simulink model "SPACE584toplevelmodel"  (R2025a)
settings: Solver=VariableStepAuto  StartTime=0.0  StopTime=10.0  RelTol=1e-3
settings Model: Creator=yvijay  LastModifiedBy=yvijay

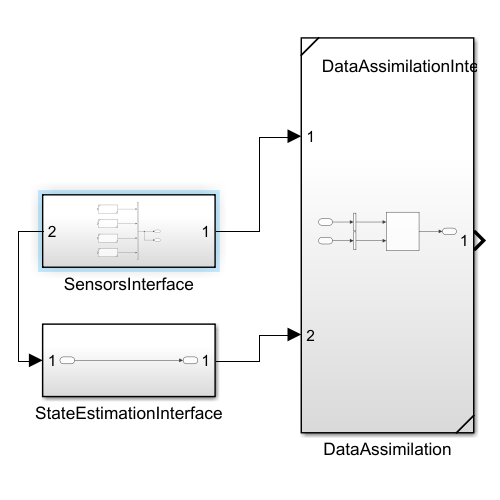
[thumbnail: Simulink's stored preview of the top-level diagram]
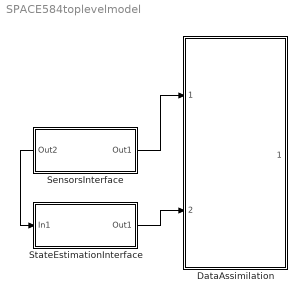
== system SPACE584toplevelmodel ==
  DataAssimilation : Subsystem  ReferencedSubsystem=DataAssimilationInterface
  SensorsInterface : Subsystem
      settings: PortSchema="{\"entries\":[{\"content\":{\"sides\":[{\"content\":{\"connectorIds\":[\"Out2\"]},\"type\":\"ConnectorPlacement.EquallySpacedRectSide\",\"uuid\":\"afeed893-a741-4527-b3e9-9d88bd0ce87b\"},{\"content\":{\"connectorIds\":[\"Out1\"],\"side\":\"RIGHT\"},\"type\":\"ConnectorPlacement.EquallySpacedRectSide\",\"uuid\":\"1d80a1de-1938-47d1-92f9-48b957537d34\"},{\"content\":{\"side\":\"TOP\"},\"type\":\"ConnectorPlacement.EquallySpacedRectSide\",\"uuid\":\"7145ccae-9960-4b20-a017-c2b7aadd2c7e\"}]},\"type\":\"ConnectorPlacement.EquallySpacedConnector\",\"uuid\":\"b07a52c2-799c-4e1c-a041-06c7de6d58f8\"}],\"packageUris\":[\"http://schema.mathworks.com/mf0/Connector/R2020b\"],\"version\":\"1.0\"}"
  StateEstimationInterface : Subsystem
  wires:
  SensorsInterface/1(Out1) -> DataAssimilation/1
  SensorsInterface/2(Out2) -> StateEstimationInterface/1(In1)
  StateEstimationInterface/1(Out1) -> DataAssimilation/2

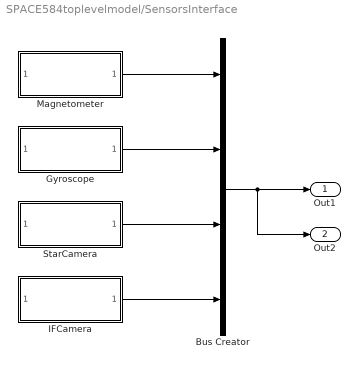
== system SPACE584toplevelmodel/SensorsInterface ==
  Bus Creator : BusCreator  Inputs=4
  Gyroscope : Subsystem  ReferencedSubsystem=Gyroscope
  IFCamera : Subsystem  ReferencedSubsystem=IFCamera
  Magnetometer : Subsystem  ReferencedSubsystem=Magnetometer
  StarCamera : Subsystem  ReferencedSubsystem=StarCamera
  Out1 : Outport
  Out2 : Outport  Port=2
  wires:
  Magnetometer/1 -> Bus Creator/1
  Gyroscope/1 -> Bus Creator/2
  StarCamera/1 -> Bus Creator/3
  IFCamera/1 -> Bus Creator/4
  Bus Creator/1 -> Out2/1, Out1/1

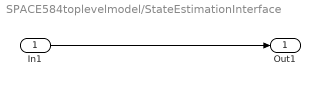
== system SPACE584toplevelmodel/StateEstimationInterface ==
  In1 : Inport
  Out1 : Outport
  wires:
  In1/1 -> Out1/1
